simulink model "UserTire"  (R2022b)
settings: Solver=ode45  StartTime=0.0  StopTime=inf  RelTol=1e-3  EnableMultiTasking=on
PreLoadFcn:
  | UserTire_params
undefined symbols (not defined in the file or in its folder): FricCoeff, Longitudinal, Side
libraries: simulink x1, CarMaker4SL x1
(part 3 of 3)

== system UserTire/CarMaker/IPG Vehicle/CarAndTrailer/Forces/Tires/UserTireFR/Side Force ==
  Alpha : Inport
  Load : Inport  Port=2
  mu : Inport  Port=3
  -Side ForceAmplify : Constant  Value=-Side.ForceAmplify
  Abs2 : Abs
  Product : Product  Inputs=3  InputSameDT=on  SaturateOnIntegerOverflow=on  OutDataTypeStr=Inherit: Same as first input
  Product3 : Product  Inputs=3  InputSameDT=on  SaturateOnIntegerOverflow=on  OutDataTypeStr=Inherit: Same as first input
  Product4 : Product  InputSameDT=on  SaturateOnIntegerOverflow=on  OutDataTypeStr=Inherit: Same as first input
  Product5 : Product  InputSameDT=on  SaturateOnIntegerOverflow=on  OutDataTypeStr=Inherit: Same as first input
  Relational Operator1 : RelationalOperator  Operator=>
  Side ForceRate : Constant  Value=Side.ForceRate
  Side FrictionRate : Constant  Value=Side.FrictionRate
  Sign : Signum
  Switch1 : Switch  Threshold=1
  F : Outport  VectorParamsAs1DForOutWhenUnconnected=off
  wires:
  mu/1 -> Product/3
  -Side ForceAmplify/1 -> Product/1
  Product/1 -> F/1
  Switch1/1 -> Product/2
  Load/1 -> Product4/1, Product3/2
  Alpha/1 -> Product3/1
  Sign/1 -> Product5/1
  Product5/1 -> Switch1/1
  Relational Operator1/1 -> Switch1/2
  Abs2/1 -> Relational Operator1/1  "absF"
  Product4/1 -> Product5/2, Relational Operator1/2  "d"
  Product3/1 -> Switch1/3, Abs2/1, Sign/1  "F"
  Side FrictionRate/1 -> Product4/2
  Side ForceRate/1 -> Product3/3

== system UserTire/CarMaker/IPG Vehicle/CarAndTrailer/Forces/Tires/UserTireFR/Side Slip Angle ==
  absvx : Inport
  vx : Inport  Port=2
  vy : Inport  Port=3
  Constant6 : Constant  Value=0.25
  Constant7 : Constant  Value=0
  Relational Operator3 : RelationalOperator  Operator=>
  Switch3 : Switch  Threshold=1
  Trigonometric Function1 : Trigonometry  Operator=atan2
  Alpha : Outport  VectorParamsAs1DForOutWhenUnconnected=off
  wires:
  Constant7/1 -> Switch3/3
  Trigonometric Function1/1 -> Switch3/1
  vy/1 -> Trigonometric Function1/1
  vx/1 -> Trigonometric Function1/2
  Switch3/1 -> Alpha/1
  absvx/1 -> Relational Operator3/1
  Relational Operator3/1 -> Switch3/2
  Constant6/1 -> Relational Operator3/2

== system UserTire/CarMaker/IPG Vehicle/CarAndTrailer/Forces/Tires/UserTireFR/Slip ==
  absvx : Inport
  vx : Inport  Port=2
  vBelt : Inport  Port=3
  Abs2 : Abs
  Constant1 : Constant  Value=0
  Constant3 : Constant  Value=0
  Constant4 : Constant  Value=0.000001
  Product1 : Product  Inputs=*/  InputSameDT=on  SaturateOnIntegerOverflow=on  OutDataTypeStr=Inherit: Same as first input
  Relational Operator1 : RelationalOperator  Operator===
  Relational Operator3 : RelationalOperator  Operator=<
  Sum1 : Sum  Inputs=-+  InputSameDT=on  SaturateOnIntegerOverflow=on  OutDataTypeStr=Inherit: Same as first input
  Switch1 : Switch  Threshold=1
  Switch3 : Switch  Threshold=1
  Slp : Outport  VectorParamsAs1DForOutWhenUnconnected=off
  wires:
  Product1/1 -> Slp/1
  Constant4/1 -> Switch1/1
  Switch1/1 -> Product1/2  "not zero"
  Constant3/1 -> Relational Operator1/1
  Relational Operator1/1 -> Switch1/2
  vBelt/1 -> Abs2/1, Sum1/2
  absvx/1 -> Switch3/1
  vx/1 -> Sum1/1
  Switch3/1 -> Switch1/3, Relational Operator1/2  "vslp"
  Abs2/1 -> Switch3/3
  Relational Operator3/1 -> Switch3/2
  Constant1/1 -> Relational Operator3/2
  Sum1/1 -> Product1/1, Relational Operator3/1  "deltav"

== system UserTire/CarMaker/IPG Vehicle/CarAndTrailer/Forces/Tires/UserTireRL/Longitudinal Force ==
  Slp : Inport
  Load : Inport  Port=2
  mu : Inport  Port=3
  Abs2 : Abs
  Longitudinal ForceRate : Constant  Value=Longitudinal.ForceRate
  Longitudinal FrictionRate : Constant  Value=Longitudinal.FrictionRate
  Product1 : Product  InputSameDT=on  SaturateOnIntegerOverflow=on  OutDataTypeStr=Inherit: Same as first input
  Product3 : Product  Inputs=3  InputSameDT=on  SaturateOnIntegerOverflow=on  OutDataTypeStr=Inherit: Same as first input
  Product4 : Product  InputSameDT=on  SaturateOnIntegerOverflow=on  OutDataTypeStr=Inherit: Same as first input
  Product5 : Product  InputSameDT=on  SaturateOnIntegerOverflow=on  OutDataTypeStr=Inherit: Same as first input
  Relational Operator1 : RelationalOperator  Operator=>
  Sign : Signum
  Switch1 : Switch  Threshold=1
  F : Outport  VectorParamsAs1DForOutWhenUnconnected=off
  wires:
  mu/1 -> Product1/2
  Product1/1 -> F/1
  Switch1/1 -> Product1/1
  Load/1 -> Product4/1, Product3/2
  Slp/1 -> Product3/1
  Sign/1 -> Product5/1
  Product5/1 -> Switch1/1
  Relational Operator1/1 -> Switch1/2
  Abs2/1 -> Relational Operator1/1  "absF"
  Product4/1 -> Product5/2, Relational Operator1/2  "d"
  Product3/1 -> Switch1/3, Abs2/1, Sign/1  "F"
  Longitudinal FrictionRate/1 -> Product4/2
  Longitudinal ForceRate/1 -> Product3/3

== system UserTire/CarMaker/IPG Vehicle/CarAndTrailer/Forces/Tires/UserTireRL/Side Force ==
  Alpha : Inport
  Load : Inport  Port=2
  mu : Inport  Port=3
  -Side ForceAmplify : Constant  Value=-Side.ForceAmplify
  Abs2 : Abs
  Product : Product  Inputs=3  InputSameDT=on  SaturateOnIntegerOverflow=on  OutDataTypeStr=Inherit: Same as first input
  Product3 : Product  Inputs=3  InputSameDT=on  SaturateOnIntegerOverflow=on  OutDataTypeStr=Inherit: Same as first input
  Product4 : Product  InputSameDT=on  SaturateOnIntegerOverflow=on  OutDataTypeStr=Inherit: Same as first input
  Product5 : Product  InputSameDT=on  SaturateOnIntegerOverflow=on  OutDataTypeStr=Inherit: Same as first input
  Relational Operator1 : RelationalOperator  Operator=>
  Side ForceRate : Constant  Value=Side.ForceRate
  Side FrictionRate : Constant  Value=Side.FrictionRate
  Sign : Signum
  Switch1 : Switch  Threshold=1
  F : Outport  VectorParamsAs1DForOutWhenUnconnected=off
  wires:
  mu/1 -> Product/3
  -Side ForceAmplify/1 -> Product/1
  Product/1 -> F/1
  Switch1/1 -> Product/2
  Load/1 -> Product4/1, Product3/2
  Alpha/1 -> Product3/1
  Sign/1 -> Product5/1
  Product5/1 -> Switch1/1
  Relational Operator1/1 -> Switch1/2
  Abs2/1 -> Relational Operator1/1  "absF"
  Product4/1 -> Product5/2, Relational Operator1/2  "d"
  Product3/1 -> Switch1/3, Abs2/1, Sign/1  "F"
  Side FrictionRate/1 -> Product4/2
  Side ForceRate/1 -> Product3/3

== system UserTire/CarMaker/IPG Vehicle/CarAndTrailer/Forces/Tires/UserTireRL/Side Slip Angle ==
  absvx : Inport
  vx : Inport  Port=2
  vy : Inport  Port=3
  Constant6 : Constant  Value=0.25
  Constant7 : Constant  Value=0
  Relational Operator3 : RelationalOperator  Operator=>
  Switch3 : Switch  Threshold=1
  Trigonometric Function1 : Trigonometry  Operator=atan2
  Alpha : Outport  VectorParamsAs1DForOutWhenUnconnected=off
  wires:
  Constant7/1 -> Switch3/3
  Trigonometric Function1/1 -> Switch3/1
  vy/1 -> Trigonometric Function1/1
  vx/1 -> Trigonometric Function1/2
  Switch3/1 -> Alpha/1
  absvx/1 -> Relational Operator3/1
  Relational Operator3/1 -> Switch3/2
  Constant6/1 -> Relational Operator3/2

== system UserTire/CarMaker/IPG Vehicle/CarAndTrailer/Forces/Tires/UserTireRL/Slip ==
  absvx : Inport
  vx : Inport  Port=2
  vBelt : Inport  Port=3
  Abs2 : Abs
  Constant1 : Constant  Value=0
  Constant3 : Constant  Value=0
  Constant4 : Constant  Value=0.000001
  Product1 : Product  Inputs=*/  InputSameDT=on  SaturateOnIntegerOverflow=on  OutDataTypeStr=Inherit: Same as first input
  Relational Operator1 : RelationalOperator  Operator===
  Relational Operator3 : RelationalOperator  Operator=<
  Sum1 : Sum  Inputs=-+  InputSameDT=on  SaturateOnIntegerOverflow=on  OutDataTypeStr=Inherit: Same as first input
  Switch1 : Switch  Threshold=1
  Switch3 : Switch  Threshold=1
  Slp : Outport  VectorParamsAs1DForOutWhenUnconnected=off
  wires:
  Product1/1 -> Slp/1
  Constant4/1 -> Switch1/1
  Switch1/1 -> Product1/2  "not zero"
  Constant3/1 -> Relational Operator1/1
  Relational Operator1/1 -> Switch1/2
  vBelt/1 -> Abs2/1, Sum1/2
  absvx/1 -> Switch3/1
  vx/1 -> Sum1/1
  Switch3/1 -> Switch1/3, Relational Operator1/2  "vslp"
  Abs2/1 -> Switch3/3
  Relational Operator3/1 -> Switch3/2
  Constant1/1 -> Relational Operator3/2
  Sum1/1 -> Product1/1, Relational Operator3/1  "deltav"

== system UserTire/CarMaker/IPG Vehicle/CarAndTrailer/Forces/Tires/UserTireRR/Longitudinal Force ==
  Slp : Inport
  Load : Inport  Port=2
  mu : Inport  Port=3
  Abs2 : Abs
  Longitudinal ForceRate : Constant  Value=Longitudinal.ForceRate
  Longitudinal FrictionRate : Constant  Value=Longitudinal.FrictionRate
  Product1 : Product  InputSameDT=on  SaturateOnIntegerOverflow=on  OutDataTypeStr=Inherit: Same as first input
  Product3 : Product  Inputs=3  InputSameDT=on  SaturateOnIntegerOverflow=on  OutDataTypeStr=Inherit: Same as first input
  Product4 : Product  InputSameDT=on  SaturateOnIntegerOverflow=on  OutDataTypeStr=Inherit: Same as first input
  Product5 : Product  InputSameDT=on  SaturateOnIntegerOverflow=on  OutDataTypeStr=Inherit: Same as first input
  Relational Operator1 : RelationalOperator  Operator=>
  Sign : Signum
  Switch1 : Switch  Threshold=1
  F : Outport  VectorParamsAs1DForOutWhenUnconnected=off
  wires:
  mu/1 -> Product1/2
  Product1/1 -> F/1
  Switch1/1 -> Product1/1
  Load/1 -> Product4/1, Product3/2
  Slp/1 -> Product3/1
  Sign/1 -> Product5/1
  Product5/1 -> Switch1/1
  Relational Operator1/1 -> Switch1/2
  Abs2/1 -> Relational Operator1/1  "absF"
  Product4/1 -> Product5/2, Relational Operator1/2  "d"
  Product3/1 -> Switch1/3, Abs2/1, Sign/1  "F"
  Longitudinal FrictionRate/1 -> Product4/2
  Longitudinal ForceRate/1 -> Product3/3

== system UserTire/CarMaker/IPG Vehicle/CarAndTrailer/Forces/Tires/UserTireRR/Side Force ==
  Alpha : Inport
  Load : Inport  Port=2
  mu : Inport  Port=3
  -Side ForceAmplify : Constant  Value=-Side.ForceAmplify
  Abs2 : Abs
  Product : Product  Inputs=3  InputSameDT=on  SaturateOnIntegerOverflow=on  OutDataTypeStr=Inherit: Same as first input
  Product3 : Product  Inputs=3  InputSameDT=on  SaturateOnIntegerOverflow=on  OutDataTypeStr=Inherit: Same as first input
  Product4 : Product  InputSameDT=on  SaturateOnIntegerOverflow=on  OutDataTypeStr=Inherit: Same as first input
  Product5 : Product  InputSameDT=on  SaturateOnIntegerOverflow=on  OutDataTypeStr=Inherit: Same as first input
  Relational Operator1 : RelationalOperator  Operator=>
  Side ForceRate : Constant  Value=Side.ForceRate
  Side FrictionRate : Constant  Value=Side.FrictionRate
  Sign : Signum
  Switch1 : Switch  Threshold=1
  F : Outport  VectorParamsAs1DForOutWhenUnconnected=off
  wires:
  mu/1 -> Product/3
  -Side ForceAmplify/1 -> Product/1
  Product/1 -> F/1
  Switch1/1 -> Product/2
  Load/1 -> Product4/1, Product3/2
  Alpha/1 -> Product3/1
  Sign/1 -> Product5/1
  Product5/1 -> Switch1/1
  Relational Operator1/1 -> Switch1/2
  Abs2/1 -> Relational Operator1/1  "absF"
  Product4/1 -> Product5/2, Relational Operator1/2  "d"
  Product3/1 -> Switch1/3, Abs2/1, Sign/1  "F"
  Side FrictionRate/1 -> Product4/2
  Side ForceRate/1 -> Product3/3

== system UserTire/CarMaker/IPG Vehicle/CarAndTrailer/Forces/Tires/UserTireRR/Side Slip Angle ==
  absvx : Inport
  vx : Inport  Port=2
  vy : Inport  Port=3
  Constant6 : Constant  Value=0.25
  Constant7 : Constant  Value=0
  Relational Operator3 : RelationalOperator  Operator=>
  Switch3 : Switch  Threshold=1
  Trigonometric Function1 : Trigonometry  Operator=atan2
  Alpha : Outport  VectorParamsAs1DForOutWhenUnconnected=off
  wires:
  Constant7/1 -> Switch3/3
  Trigonometric Function1/1 -> Switch3/1
  vy/1 -> Trigonometric Function1/1
  vx/1 -> Trigonometric Function1/2
  Switch3/1 -> Alpha/1
  absvx/1 -> Relational Operator3/1
  Relational Operator3/1 -> Switch3/2
  Constant6/1 -> Relational Operator3/2

== system UserTire/CarMaker/IPG Vehicle/CarAndTrailer/Forces/Tires/UserTireRR/Slip ==
  absvx : Inport
  vx : Inport  Port=2
  vBelt : Inport  Port=3
  Abs2 : Abs
  Constant1 : Constant  Value=0
  Constant3 : Constant  Value=0
  Constant4 : Constant  Value=0.000001
  Product1 : Product  Inputs=*/  InputSameDT=on  SaturateOnIntegerOverflow=on  OutDataTypeStr=Inherit: Same as first input
  Relational Operator1 : RelationalOperator  Operator===
  Relational Operator3 : RelationalOperator  Operator=<
  Sum1 : Sum  Inputs=-+  InputSameDT=on  SaturateOnIntegerOverflow=on  OutDataTypeStr=Inherit: Same as first input
  Switch1 : Switch  Threshold=1
  Switch3 : Switch  Threshold=1
  Slp : Outport  VectorParamsAs1DForOutWhenUnconnected=off
  wires:
  Product1/1 -> Slp/1
  Constant4/1 -> Switch1/1
  Switch1/1 -> Product1/2  "not zero"
  Constant3/1 -> Relational Operator1/1
  Relational Operator1/1 -> Switch1/2
  vBelt/1 -> Abs2/1, Sum1/2
  absvx/1 -> Switch3/1
  vx/1 -> Sum1/1
  Switch3/1 -> Switch1/3, Relational Operator1/2  "vslp"
  Abs2/1 -> Switch3/3
  Relational Operator3/1 -> Switch3/2
  Constant1/1 -> Relational Operator3/2
  Sum1/1 -> Product1/1, Relational Operator3/1  "deltav"
